simulink model "ProcessFlowRateModel"  (Simulink 7.9)
settings: Solver=VariableStepDiscrete  StartTime=0.0  StopTime=100.0  RelTol=1e-3
libraries: simeventslib x9
(part 2 of 2)

== matlab function CartonPickFromPalletStore/Calculate_INFlow/Calculate_INFlow ==
  data: UoH input double; INFlow_return output double; Quantity input double; INFlow input double
function INFlow_return  = Calculate_INFlow(UoH, Quantity, INFlow)
%#codegen

INFlow_return = INFlow;


if eq(UoH, 0) == 0
%test if parameters are initialized

    INFlow_return(UoH) = INFlow(UoH) + Quantity;
end

== matlab function CartonPickFromPalletStore/Calculate_OUTFlow/Calculate_OUTFlow ==
  data: UoH input double; OUTFlow_return output double; Quantity input double; OUTFlow input double
function OUTFlow_return  = Calculate_OUTFlow(UoH, Quantity, OUTFlow)
%#codegen

OUTFlow_return = OUTFlow;


if eq(UoH, 0) == 0
%test if parameters are initialized

    OUTFlow_return(UoH) = OUTFlow(UoH) + Quantity;
end

== matlab function CartonPickFromPalletStore/CartonPick/Pick_CycleTime/MATLAB Function ==
  data: Quantity input double; PickCycleTime output double
function PickCycleTime = fcn(Quantity)
%#codegen

coder.extrinsic('normrnd');
PickCycleTime = zeros(1, 'double');

Pick_Mean = Quantity*30;
Pick_StdDev = Quantity*5;

PickCycleTime = normrnd(Pick_Mean, sqrt(Pick_StdDev));
